simulink library "uavsimblockset_vbody2vNED"  (Simulink 8.4)
settings: Solver=ode45  StartTime=0.0  StopTime=10.0  RelTol=1e-3
settings Model: Creator=mstolle  LastModifiedBy=j.bolting

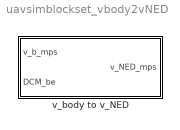
== system uavsimblockset_vbody2vNED ==
  v_body to v_NED : Subsystem

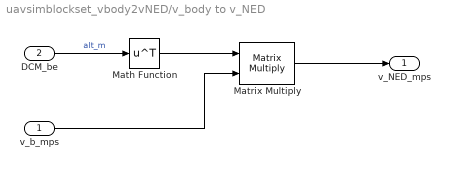
== system uavsimblockset_vbody2vNED/v_body to v_NED ==
  v_b_mps : Inport
  DCM_be : Inport  Port=2
  Math Function : Math  Operator=transpose  SaturateOnIntegerOverflow=on
  Matrix Multiply : Product  Multiplication=Matrix(*)
  v_NED_mps : Outport
  wires:
  Matrix Multiply/1 -> v_NED_mps/1
  v_b_mps/1 -> Matrix Multiply/2
  Math Function/1 -> Matrix Multiply/1
  DCM_be/1 -> Math Function/1  "alt_m"
